simulink model "Commander_Stabilizer_Qdrone_wTrajTEMP"  (R2019a)
settings: Solver=ode2  StartTime=0.0  StopTime=inf  FixedStep=0.001  RelTol=1e-3  EnableMultiTasking=on
InitFcn:
  | set_param(gcs, 'ZoomFactor','FitSystem')
model workspace (MAT data in the model file):
  target_system = 1
undefined symbols (not defined in the file or in its folder): acc_calib, HIL
libraries: quarc_library x50, simulink x20, control_library x13, estimation_library x7
(part 3 of 3)

== matlab function Commander_Stabilizer_Qdrone_wTrajTEMP/Inner loop controller /inner loop MRFT subsytem/MRFT_NEW 1/MATLAB Function ==
  settings: updateMethod=DISCRETE
  data: err input; output output; beta input; h input; no_switch_delay_in_s input; num_of_peak_conf_samples input; sim_time input; e_max_o output; e_min_o output; sw_max_o output; sw_min_o output
% MRFT algorithm with false switching prevention mechanism
% June 2020
% Coded By M. Chehadeh, Khalifa University
function [output,e_max_o,e_min_o,sw_max_o,sw_min_o]  = MRFT(err,beta,h,no_switch_delay_in_s,num_of_peak_conf_samples,sim_time)
persistent switch_time;
persistent last_output;
persistent e_max;
persistent e_min;
persistent has_reached_min;
persistent has_reached_max;
persistent peak_conf_counter;
mode_of_operation=1;
% mode_of_operation=0 take last e_max or e_min
% mode_of_operation=1 take current e_max or e_min and mirror it

output=0;
e_max_o=0;
e_min_o=0;
sw_max_o=0;
sw_min_o=0;
if isempty(switch_time)
    switch_time = sim_time;
    peak_conf_counter=0;
    e_max=0;
    e_min=0;
    if (err>0)
        has_reached_max=true;
        has_reached_min=false;
        last_output=h;
    else
        has_reached_max=false;
        has_reached_min=true;
        last_output=-h;
    end
    output=last_output;
    return;  
end
output=last_output;
if (sim_time-switch_time<=no_switch_delay_in_s)
    e_min_o=e_min;
    e_max_o=e_max;
    return;
end

if (last_output<0)
    if (err<e_min)
        e_min=err;
        peak_conf_counter=0;
    else
        peak_conf_counter=peak_conf_counter+1;
        if (peak_conf_counter>=num_of_peak_conf_samples)
            has_reached_min=true;
            peak_conf_counter=0;
        end
        e_max=err;
    end
    if (mode_of_operation==0)
        sw_min=((e_max-e_min)/2)+e_min+beta*((e_max-e_min)/2);
    elseif (mode_of_operation==1)
        e_max_star=-e_min;
        sw_min=((e_max_star-e_min)/2)+e_min+beta*((e_max_star-e_min)/2);
    end
    sw_min_o=sw_min;
    if (has_reached_min)
        if (err>sw_min)
            output=h;
            switch_time=sim_time;
            has_reached_min=false;
        else
            output=last_output;
        end
    end
else
    if (err>e_max)
        e_max=err;
        peak_conf_counter=0;
    else
        peak_conf_counter=peak_conf_counter+1;
        if (peak_conf_counter>=num_of_peak_conf_samples)
            has_reached_max=true;
            peak_conf_counter=0;
        end
        e_min=err;
    end
    if (mode_of_operation==0)
        sw_max=e_max-((e_max-e_min)/2)-(beta*((e_max-e_min)/2));
    elseif (mode_of_operation==1)
        e_min_star=-e_max;
        sw_max=e_max-((e_max-e_min_star)/2)-(beta*((e_max-e_min_star)/2));
    end    
    sw_max_o=sw_max;
    if (has_reached_max)
        if (err<sw_max)
            output=-h;
            switch_time=sim_time;
            has_reached_max=false;
        else
            output=last_output;
        end
    end
end
e_min_o=e_min;
e_max_o=e_max;
last_output=output;

== matlab function Commander_Stabilizer_Qdrone_wTrajTEMP/Outer loop/MATLAB Function ==
  data: FSM_state input; HF_smoothed_commands output; HF_desired_state input; HF_current_state input; safety_threshold input; height_signals output
function [HF_smoothed_commands, height_signals] = fcn(FSM_state, HF_desired_state, HF_current_state, safety_threshold)

HF_desired_state = min(HF_desired_state, safety_threshold);
HF_desired_state = max(HF_desired_state, -safety_threshold);

HF_smoothed_commands = HF_desired_state;
switch FSM_state
    case 1
        HF_smoothed_commands = HF_current_state;
    case 2
        HF_smoothed_commands = HF_current_state;
    case 3
        delta_move = (HF_desired_state - HF_current_state);
        delta_move_norm = norm(delta_move);
        if delta_move_norm>0.2
            delta_move = 0.2 * delta_move / delta_move_norm;
        end
        HF_smoothed_commands = HF_current_state + delta_move;
    case 4
        delta_move = (HF_desired_state - HF_current_state);
        delta_move_norm = norm(delta_move);
        if delta_move_norm>0.2
            delta_move = 0.2 * delta_move / delta_move_norm;
        end
        HF_smoothed_commands = HF_current_state + delta_move;
    case 5
        HF_smoothed_commands = HF_desired_state;%HF_current_state + 0.2*(HF_desired_state - HF_current_state) / norm(HF_desired_state - HF_current_state);
    case 6
        HF_low_desired_state = HF_current_state;
        HF_low_desired_state(3) = 0.1;        
        delta_move = (HF_low_desired_state - HF_current_state);
        delta_move_norm = norm(delta_move);
        if delta_move_norm>0.1
            delta_move = 0.1 * delta_move / delta_move_norm;
        end
        HF_smoothed_commands = HF_current_state + delta_move;
    case 7
        HF_low_desired_state = HF_current_state;
        HF_low_desired_state(3) = 0.1;        
        delta_move = (HF_low_desired_state - HF_current_state);
        delta_move_norm = norm(delta_move);
        if delta_move_norm>0.2
            delta_move = 0.2 * delta_move / delta_move_norm;
        end
        HF_smoothed_commands = HF_current_state + delta_move;
    case 8
        
        HF_low_desired_state = HF_current_state;
        HF_low_desired_state(3) = 0.1;        
        delta_move = (HF_low_desired_state - HF_current_state);
        delta_move_norm = norm(delta_move);
        if delta_move_norm>0.2
            delta_move = 0.2 * delta_move / delta_move_norm;
        end
        HF_smoothed_commands = HF_current_state + delta_move;
    case 9        
        HF_low_desired_state = HF_desired_state;
        HF_low_desired_state(3) = 0.1;        
        delta_move = (HF_low_desired_state - HF_current_state);
        delta_move_norm = norm(delta_move);
        if delta_move_norm>0.2
            delta_move = 0.2 * delta_move / delta_move_norm;
        end
        HF_smoothed_commands = HF_current_state + delta_move;
end

height_signals = [HF_smoothed_commands(3), HF_current_state(3), safety_threshold(3), HF_desired_state(3)]';

== matlab function Commander_Stabilizer_Qdrone_wTrajTEMP/motor command mapper/Set commands/Red - Low Voltage Green - Armed Blue - Disarmed/MATLAB Function LED Color Assignment ==
  data: arm input; value output; low_battery input
function value = fcn(arm, low_battery)

if low_battery
    value = 1;
elseif arm
    value = 2;
else 
    value = 3;
end

== matlab function Commander_Stabilizer_Qdrone_wTrajTEMP/logic/FSM MONITOR/STATE MACHINE LOGIC ==
  data: E_Abort output; isArm output; pt_ARM_to_TAKEOFF_THROTTLE output; pt_TAKE_OFF_HEIGHT_TO_AUTOLAND output; pt_FLIGHT_TO_AUTOLAND output; current_state input; initializing input; health_issue input; peripheral input; low_battery input; trigger_1 input; trigger_2 input; E_abort input; net_throttle_at_trim input; net_throttle_close_to_zero input; ctrl_throttle_close_to_zero input; take_off_successful input; flying_too_low input; flying_too_high input; close_to_ground input; pt_TAKEOFF_THROTTLE_TO_TAKEOFF_HEIGHT output; pt_TAKE_OFF_HEIGHT_TO_FLIGHT output; pt_AUTOLAND_TO_DISABLE output; pt_EMERGENCY_STOP_TO_DISABLE output; pt_EMERGENCY_ABORT_TO_DISABLE output; Error output; stop_model output; sensor_failed input
function [E_Abort, isArm, pt_ARM_to_TAKEOFF_THROTTLE, pt_TAKE_OFF_HEIGHT_TO_AUTOLAND, pt_FLIGHT_TO_AUTOLAND, pt_TAKEOFF_THROTTLE_TO_TAKEOFF_HEIGHT, pt_TAKE_OFF_HEIGHT_TO_FLIGHT, pt_AUTOLAND_TO_DISABLE, pt_EMERGENCY_STOP_TO_DISABLE, pt_EMERGENCY_ABORT_TO_DISABLE, Error, stop_model]...
    = SM_logic(current_state, initializing, health_issue, peripheral, low_battery, trigger_1, trigger_2, E_abort,...
    net_throttle_at_trim, net_throttle_close_to_zero, ctrl_throttle_close_to_zero, take_off_successful, flying_too_low, flying_too_high, close_to_ground, sensor_failed)

% Programmatic Logic Block
%
% Logic for the FSM is generated here based on a variety of signals.
% Mostly, logic to programmatically trigger the transition to either a 
% natural next state, or an Error state, is generated here.
%
% v2.1 - 4th October, 2018
%
% INPUTS:
% -------
% current_state = previous state of the FSM-------------------------------------------------- (#)         [1]
% initializing = signal representing that the system is initializing (first 5s + buffer)- - - (bool)      [1]
% comm = communication signal representing MAVLINK connection-------------------------------- (bool)      [1]
% peripheral = signal representing joystick and optitrack connection- - - - - - - - - - - - - (bool)      [2]
% low_battery = signal representing low battery---------------------------------------------- (bool)      [1]
% trigger_1 = trigger representing ARM/DISARM - - - - - - - - - - - - - - - - - - - - - - - - (bool)      [1]
% trigger_2 = trigger representing TAKEOFF/AUTOLAND------------------------------------------ (bool)      [1]
% motors_not_spinning = signal representing the motors not spinning - - - - - - - - - - - - - (bool)      [1]
% net_throttle_at_trim = trim throttle for the application drone ---------------------------- (bool)      [1]
% net_throttle_close_to_zero = net throttle is close to zero in emergency stop mode - - - - - (bool)      [1]
% ctrl_throttle_close_to_zero = ctrl throttle is close to zero in emergency stop mode - - - - (bool)      [1]
% take_off_successful = signal representing whether drone has taken-off successfully -------- (bool)      [1]
% flying_too_low = signal representing whether the drone's height is below threshold and cmd- (bool)      [1]
% flying_too_high = signal representing whether the drone's height is above threshold-------- (bool)      [1]
% close_to_ground = signal representing whether the drone is close to the ground to autoland- (bool)      [1]
% 
% OUTPUTS:
% --------
% Error = Whether an Error is issued or not                                                             (bool)    [1]
% E_Abort = fed through for ease of understanding flow (see STATE MACHINE TRANSITION BLOCK)             (bool)    [1]
% isArm = programmatic transition state                                                                 (bool)    [1]
% pt_ARM_to_TAKEOFF_THROTTLE = programmatic transition state BEGIN_STATE_TO_FINAL_STATE                 (bool)    [1]
% pt_TAKEOFF_THROTTLE_TO_TAKEOFF_HEIGHT = programmatic transition state BEGIN_STATE_TO_FINAL_STATE      (bool)    [1]
% pt_TAKE_OFF_HEIGHT_TO_AUTOLAND = programmatic transition state BEGIN_STATE_TO_FINAL_STATE             (bool)    [1]
% pt_TAKEOFF_THROTTLE_TO_TAKEOFF_HEIGHT = programmatic transition state BEGIN_STATE_TO_FINAL_STATE      (bool)    [1]
% pt_TAKE_OFF_HEIGHT_TO_FLIGHT = programmatic transition state BEGIN_STATE_TO_FINAL_STATE               (bool)    [1]
% pt_AUTOLAND_TO_DISABLE = programmatic transition state BEGIN_STATE_TO_FINAL_STATE                     (bool)    [1]
% pt_EMERGENCY_STOP_TO_DISABLE = programmatic transition state BEGIN_STATE_TO_FINAL_STATE               (bool)    [1]
% pt_EMERGENCY_ABORT_TO_DISABLE = programmatic transition state BEGIN_STATE_TO_FINAL_STATE              (bool)    [1]
% stop_model = STOP THE MODEL AFTER                                                                     (bool)    [1]

Error = 0;
E_Abort = E_abort;
isArm = false;
pt_ARM_to_TAKEOFF_THROTTLE = false;
pt_TAKEOFF_THROTTLE_TO_TAKEOFF_HEIGHT = false;
pt_TAKE_OFF_HEIGHT_TO_AUTOLAND = false;
pt_TAKE_OFF_HEIGHT_TO_FLIGHT = false;
pt_FLIGHT_TO_AUTOLAND = false;
pt_AUTOLAND_TO_DISABLE = false;
pt_EMERGENCY_STOP_TO_DISABLE = false;
pt_EMERGENCY_ABORT_TO_DISABLE = false;
stop_model = 0;

switch current_state
    %---------------------------------------------------------------------%
    case 1 % IDLE STATE
        if (health_issue)||... % mavlink issue
           (peripheral(1))||... % joystick issue
           (peripheral(2))||... % optitrack issue
           ((trigger_1)&&(initializing))||... % armed while initializing
           (trigger_2)||... % tried to takeoff
           (sensor_failed)||... % if sensor (IMU) failure is detected on drone stabilizer
           (~ctrl_throttle_close_to_zero)||... % if throttle isn't at zero, don't arm
           (low_battery) % low battery
           %----------------------------------------%
            Error = 1;
        elseif trigger_1 % user arms
            isArm = true;
        end
    %---------------------------------------------------------------------%    
    case 2 % ARMED STATE
        isArm = trigger_1;
        if (health_issue)||... % mavlink issue
           (peripheral(1))||... % joystick issue
           (peripheral(2))||... % optitrack issue
           (low_battery)||... % low battery
           (~ctrl_throttle_close_to_zero)||... % if throttle isn't at zero, don't arm
           (sensor_failed) % if sensor (IMU) failure is detected on drone stabilizer
           %----------------------------------------%
            Error = 1;
        elseif trigger_1 && trigger_2
            pt_ARM_to_TAKEOFF_THROTTLE = true;
        end        
    %---------------------------------------------------------------------%
    case 3 % TAKEOFF_THROTTLE STATE
        if (health_issue)||... % mavlink issue
           (peripheral(1))||... % joystick issue
           (peripheral(2))||... % optitrack issue
           (low_battery)||... % low battery
           (~trigger_1)||... % user disarms
           (~trigger_2)||... % user commands auto-land before drone starts taking off
           (sensor_failed)%||... % if sensor (IMU) failure is detected on drone stabilizer
           %(~ctrl_throttle_close_to_zero) % if throttle isn't at zero, don't arm
           %----------------------------------------%
            Error = 1;
        elseif net_throttle_at_trim
            pt_TAKEOFF_THROTTLE_TO_TAKEOFF_HEIGHT = true;
        end
    %---------------------------------------------------------------------%
    case 4 % TAKEOFF_HEIGHT STATE
        if (health_issue)||... % mavlink issue
           (peripheral(1))||... % joystick issue
           (peripheral(2))||... % optitrack issue
           (~trigger_1)||... % user disarms
           (sensor_failed)||... % if sensor (IMU) failure is detected on drone stabilizer
           (flying_too_high)
           %(flying_too_low)||... % current height is below safety threshold but 
           %...                   % commanded height is not
           
            %----------------------------------------%
            Error = 1;
        elseif (~trigger_2)||low_battery
            pt_TAKE_OFF_HEIGHT_TO_AUTOLAND = true;
        elseif take_off_successful
            pt_TAKE_OFF_HEIGHT_TO_FLIGHT = true;
        end
    %---------------------------------------------------------------------%
    case 5 % FLIGHT STATE
        if (health_issue)||... % mavlink issue
           (peripheral(1))||... % joystick issue
           (peripheral(2))||... % optitrack issue
           (~trigger_1)||... % user disarms
           (flying_too_low)||... % current height is below safety threshold but 
           ...                   % commanded height is not
           (sensor_failed)||... % if sensor (IMU) failure is detected on drone stabilizer
           (flying_too_high) % flying above safety margin (w.r.t optitrack)
           %----------------------------------------%
            Error = 1;
        elseif (~trigger_2)||low_battery
            pt_FLIGHT_TO_AUTOLAND = true;
        end
    %---------------------------------------------------------------------%
    case 6 % AUTOLAND STATE
        if (health_issue)||... % mavlink issue
           (peripheral(1))||... % joystick issue
           (peripheral(2))||... % optitrack issue
           (~trigger_1)||... % user disarms
           (trigger_2)||... % user tries to takeoff while landing
           (sensor_failed)||... % if sensor (IMU) failure is detected on drone stabilizer
           (flying_too_high) % flying above safety margin (w.r.t optitrack)
           %----------------------------------------%
            Error = 1;
        elseif close_to_ground 
            pt_AUTOLAND_TO_DISABLE = true;
        end
    %---------------------------------------------------------------------%
    case 7 % EMERGENCY LAND STATE
        if net_throttle_close_to_zero 
            pt_EMERGENCY_STOP_TO_DISABLE = true;
        end
    %---------------------------------------------------------------------%
    case 8 % EMERGENCY ABORT STATE
        pt_EMERGENCY_ABORT_TO_DISABLE = true;
    %---------------------------------------------------------------------%
    case 9
        % Stop the model.
        stop_model = 1;
end

== matlab function Commander_Stabilizer_Qdrone_wTrajTEMP/logic/FSM MONITOR/STATE MACHINE TRANSITION ==
  data: current_state input; E_Abort input; isArm input; pt_ARM_to_TAKEOFF_THROTTLE input; pt_TAKE_OFF_HEIGHT_TO_AUTOLAND input; pt_FLIGHT_TO_AUTOLAND input; Next_state output; pt_TAKEOFF_THROTTLE_TO_TAKEOFF_HEIGHT input; pt_TAKE_OFF_HEIGHT_TO_FLIGHT input; pt_AUTOLAND_TO_DISABLE input; pt_EMERGENCY_STOP_TO_DISABLE input; pt_EMERGENCY_ABORT_TO_DISABLE input; Error input
function Next_state = SM_transition(current_state, E_Abort, isArm, pt_ARM_to_TAKEOFF_THROTTLE, pt_TAKE_OFF_HEIGHT_TO_AUTOLAND, pt_FLIGHT_TO_AUTOLAND, pt_TAKEOFF_THROTTLE_TO_TAKEOFF_HEIGHT, pt_TAKE_OFF_HEIGHT_TO_FLIGHT, pt_AUTOLAND_TO_DISABLE, pt_EMERGENCY_STOP_TO_DISABLE, pt_EMERGENCY_ABORT_TO_DISABLE, Error)

% Programmatic Transition Block
%
% FINITE STATE MACHINE (FSM) with 9 states as described below, transitioning based on the 
% values of the isArm, transition signals, Error, and E_Abort
%
% v2.1 - 4th October, 2018
%
% INPUTS:
% ------
% current_state = Current state of the FSM        (#)     [1]
% E_Abort                                         (bool)  [1]
% isArm                                           (bool)  [1]
% pt_ARM_TO_TAKEOFF_THROTTLE                      (bool)  [1]
% pt_TAKE_OFF_HEIGHT_TO_AUTOLAND                  (bool)  [1]
% pt_FLIGHT_TO_AUTOLAND                           (bool)  [1]
% pt_TAKEOFF_THROTTLE_TO_TAKEOFF_HEIGHT           (bool)  [1]
% pt_TAKE_OFF_HEIGHT_TO_FLIGHT                    (bool)  [1]
% pt_AUTOLAND_TO_DISABLE                          (bool)  [1]
% pt_EMERGENCY_STOP_TO_DISABLE                    (bool)  [1]
% pt_EMERGENCY_ABORT_TO_DISABLE                   (bool)  [1]
% Error                                           (bool)  [1]
%
% OUTPUT:
% -------
% Next_state = Next state of the FSM              (#)     [1]

Next_state = double(0);
switch current_state
%-------------------------------------------------------------------------%
    case 1 % IDLE STATE
        if E_Abort
            Next_state = 8; % GOTO EMERGENCY ABORT STATE
        elseif Error
            Next_state = 7; % GOTO EMERGENCY STOP STATE
        elseif isArm
            Next_state = 2; % GOTO ARMED STATE
        else
            Next_state = 1; % STAY IN IDLE STATE
        end
%-------------------------------------------------------------------------%
    case 2 % ARMED STATE
        if E_Abort
            Next_state = 8; % GOTO EMERGENCY ABORT STATE
        elseif Error
            Next_state = 7; % GOTO EMERGENCY STOP STATE
        elseif ~isArm
            Next_state = 1; % GOTO IDLE STATE
        elseif pt_ARM_to_TAKEOFF_THROTTLE
            Next_state = 3; % GOTO TAKEOFF_THROTTLE STATE 
        else
            Next_state = 2; % STAY IN ARMED STATE
        end
%-------------------------------------------------------------------------%
    case 3 % TAKEOFF_THROTTLE STATE
        if E_Abort
            Next_state = 8; % GOTO EMERGENCY ABORT STATE
        elseif Error
            Next_state = 7; % GOTO EMERGENCY STOP STATE
        elseif pt_TAKEOFF_THROTTLE_TO_TAKEOFF_HEIGHT
            Next_state = 4; % GOTO TAKEOFF_HEIGHT STATE
        else
            Next_state = 3; % STAY IN TAKEOFF_THROTTLE STATE
        end
%-------------------------------------------------------------------------%
    case 4 % TAKEOFF_HEIGHT STATE
        if E_Abort
            Next_state = 8; % GOTO EMERGENCY ABORT STATE
        elseif Error
            Next_state = 7; % GOTO EMERGENCY STOP STATE
        elseif pt_TAKE_OFF_HEIGHT_TO_AUTOLAND
            Next_state = 6;
        elseif pt_TAKE_OFF_HEIGHT_TO_FLIGHT
            Next_state = 5; % GOTO FLIGHT STATE
        else
            Next_state = 4; % STAY IN TAKEOFF_HEIGHT STATE
        end
%-------------------------------------------------------------------------%
    case 5 % FLIGHT STATE
        if E_Abort
            Next_state = 8; % GOTO EMERGENCY ABORT STATE
        elseif Error
            Next_state = 7; % GOTO EMERGENCY STOP STATE
        elseif pt_FLIGHT_TO_AUTOLAND
            Next_state = 6; % GOTO AUTO_LAND STATE
        else
            Next_state = 5; % STAY IN FLIGHT STATE
        end
%-------------------------------------------------------------------------%       
    case 6 % AUTO_LAND STATE
        if E_Abort
            Next_state = 8; % GOTO EMERGENCY ABORT STATE
        elseif Error
            Next_state = 7; % GOTO EMERGENCY STOP STATE
        elseif pt_AUTOLAND_TO_DISABLE
            Next_state = 9; % GOTO DISABLE STATE
        else
            Next_state = 6; % STAY IN AUTO_LAND STATE
        end
%-------------------------------------------------------------------------%
    case 7 % EMERGENCY STOP STATE
        if E_Abort
            Next_state = 8; % GOTO EMERGENCY ABORT STATE
        elseif pt_EMERGENCY_STOP_TO_DISABLE
            Next_state = 9; % GOTO DISABLE STATE
        else
            Next_state = 7; % STAY IN EMERGENCY STOP STATE
        end
%-------------------------------------------------------------------------%
    case 8 % EMERGENCY ABORT
        if pt_EMERGENCY_ABORT_TO_DISABLE
            Next_state = 9; % GOTO DISABLE STATE
        else 
            Next_state = 8; % STAY IN EMERGENCY ABORT STATE
        end
%-------------------------------------------------------------------------%    
    case 9 % DISABLE
        Next_state = 9; % Always stay in DISABLE state if you are here    
end

== matlab function Commander_Stabilizer_Qdrone_wTrajTEMP/Pull Detector1/MATLAB Function ==
  settings: updateMethod=DISCRETE  sampleTime=0.001
  data: error_z input; acc_x input; acc_y input; acc_z input; roll input; pitch input; yaw input; detection_output output
function detection_output  = LSTM(error_z, acc_x, acc_y, acc_z, roll, pitch, yaw)

persistent drone_handover_model
persistent p_01_h_t
persistent p_01_c_t
persistent p_03_h_t
persistent p_03_c_t
persistent scaling_params
persistent buffer
persistent counter
persistent clean_detection

downsample_by = 5;

if isempty(drone_handover_model)
    drone_handover_model = coder.load('Model_2f_norm/drone_handover_model.mat');
    scaling_params = coder.load('Model_2f_norm/Scaling.mat');
    p_01_h_t = single(zeros(1,200));
    p_01_c_t = single(randn(1,200)/10);
    p_03_h_t = single(zeros(1,100));
    p_03_c_t = single(randn(1,100)/10);
    buffer = single(zeros(7,downsample_by));
    counter = 1;
    clean_detection = 0;
end

buffer(1,counter) = error_z;
buffer(2,counter) = acc_x;
buffer(3,counter) = acc_y;
buffer(4,counter) = acc_z;
buffer(5,counter) = roll;
buffer(6,counter) = pitch;
buffer(7,counter) = yaw;

if counter == 5
    counter = 1;
    error_z = mean(buffer(1,:));
    acc_x = mean(buffer(2,:));
    acc_y = mean(buffer(3,:));
    acc_z = mean(buffer(4,:));
    roll = mean(buffer(5,:));
    pitch = mean(buffer(6,:));
    yaw = mean(buffer(7,:));
    % 
    [acc_x_inertial, acc_y_inertial, acc_z_inertial] = R_B2I(roll, pitch, yaw, acc_x, acc_y, acc_z);
    % 
    l2_norm_acc_inertial = sqrt(acc_x_inertial.^2 + acc_y_inertial.^2);
    % 
    % [ori_body_x, ori_body_y, ori_body_z] = R_I2B(roll, pitch, yaw, 0, 0, 1);
    % 
%     l2_norm_ori = sqrt(ori_body_x.^2 + ori_body_y.^2);
%     % 
%     acc_dir = atan2(acc_y_inertial, acc_x_inertial);
%     ori_dir = atan2(ori_body_y, ori_body_x);
%     
%     if abs(acc_dir - ori_dir) <= pi
%         dist_acc_ori = abs(acc_dir - ori_dir);
%     else
%         dist_acc_ori = 2*pi - abs(acc_dir - ori_dir);
%     end
    
    % %%Scaling
    % % X_std = (X - X.min(axis=0)) / (X.max(axis=0) - X.min(axis=0))
    error_z = (error_z - scaling_params.data_Z_params(1)) / (scaling_params.data_Z_params(2)-scaling_params.data_Z_params(1));
    error_z = error_z * 2 - 1;
    l2_norm_acc_inertial = (l2_norm_acc_inertial  - scaling_params.data_L2_norm_inertial_params(1)) / (scaling_params.data_L2_norm_inertial_params(2)-scaling_params.data_L2_norm_inertial_params(1));
    l2_norm_acc_inertial = l2_norm_acc_inertial * 2 - 1;
    %     l2_norm_ori = (l2_norm_ori - scaling_params.data_L2_norm_ori_params(1)) / (scaling_params.data_L2_norm_ori_params(2)-scaling_params.data_L2_norm_ori_params(1));
%     dist_acc_ori = (dist_acc_ori - scaling_params.data_dist_acc_ori_params(1)) / (scaling_params.data_dist_acc_ori_params(2)-scaling_params.data_dist_acc_ori_params(1));
    % 

    input_data = [error_z l2_norm_acc_inertial];

    [detection, p_01_c_t, p_01_h_t, p_03_c_t, p_03_h_t] = model_classify(input_data, ...
                                                                         drone_handover_model, ...
                                                                         p_01_c_t, ...
                                                                         p_01_h_t, ...
                                                                         p_03_c_t, ...
                                                                         p_03_h_t);
                                                                     
    clean_detection = clean(detection, 0.5);
%     clean_detection = double(detection);
end

counter = counter + 1;

% dist_acc_ori_out = dist_acc_ori;
% l2_norm_ori_out = l2_norm_ori;
% l2_norm_acc_out = l2_norm_acc_inertial;
detection_output = double(clean_detection);

% function [detection_output, error_output, l2_output] = LSTM_offline(error_z_, l2_norm_acc_inertial_)
% 
% persistent drone_handover_model
% persistent p_01_h_t
% persistent p_01_c_t
% persistent p_03_h_t
% persistent p_03_c_t
% persistent scaling_params
% persistent buffer
% persistent counter
% persistent clean_detection
% 
% downsample_by = 5;
% 
% if isempty(drone_handover_model)
%     drone_handover_model = coder.load('Model_2f_norm/drone_handover_model.mat');
%     p_01_h_t = single(zeros(1,200));
%     p_01_c_t = single(randn(1,200)/10);
%     p_03_h_t = single(zeros(1,100));
%     p_03_c_t = single(randn(1,100)/10);
%     buffer = single(zeros(7,downsample_by));
%     counter = 1;
%     clean_detection = 0;
% end
% 
% 
% input_data = [error_z_ l2_norm_acc_inertial_];
% 
% [detection, p_01_c_t, p_01_h_t, p_03_c_t, p_03_h_t] = model_classify(input_data, ...
%                                                                      drone_handover_model, ...
%                                                                      p_01_c_t, ...
%                                                                      p_01_h_t, ...
%                                                                      p_03_c_t, ...
%                                                                      p_03_h_t);
% 
% clean_detection = clean(detection, 0.5);
% 
% error_output = error_z_;
% l2_output = l2_norm_acc_inertial_;
% detection_output = double(clean_detection);

== matlab function Commander_Stabilizer_Qdrone_wTrajTEMP/Pull Detector1/MATLAB Function1 ==
  settings: updateMethod=DISCRETE  sampleTime=0.001
  data: u input; y output; threshold input
function y = prediction_filter(u, threshold)

persistent counter_ones
persistent counter_zeros
persistent pull_detected
persistent prev_u

if isempty(counter_ones)
    counter_ones = 0;
    counter_zeros = 0;
    prev_u = 0;
end

if u == 1
    counter_ones = counter_ones + 1;
else
    counter_zeros = counter_zeros + 1;     
end

if prev_u == 0 && u == 1
    counter_zeros = 0;
end

if counter_ones > threshold && counter_zeros < threshold
    pull_detected = 1;
else
    pull_detected = 0;
end

if counter_zeros >= threshold
    counter_ones = 0;
end

prev_u = double(u);
y = pull_detected;

== matlab function Commander_Stabilizer_Qdrone_wTrajTEMP/Inner loop controller /inner loop MRFT subsytem/MRFT_NEW /MATLAB Function ==
  settings: updateMethod=DISCRETE
  data: err input; output output; beta input; h input; no_switch_delay_in_s input; num_of_peak_conf_samples input; sim_time input; e_max_o output; e_min_o output; sw_max_o output; sw_min_o output
% MRFT algorithm with false switching prevention mechanism
% June 2020
% Coded By M. Chehadeh, Khalifa University
function [output,e_max_o,e_min_o,sw_max_o,sw_min_o]  = MRFT(err,beta,h,no_switch_delay_in_s,num_of_peak_conf_samples,sim_time)
persistent switch_time;
persistent last_output;
persistent e_max;
persistent e_min;
persistent has_reached_min;
persistent has_reached_max;
persistent peak_conf_counter;
mode_of_operation=1;
% mode_of_operation=0 take last e_max or e_min
% mode_of_operation=1 take current e_max or e_min and mirror it

output=0;
e_max_o=0;
e_min_o=0;
sw_max_o=0;
sw_min_o=0;
if isempty(switch_time)
    switch_time = sim_time;
    peak_conf_counter=0;
    e_max=0;
    e_min=0;
    if (err>0)
        has_reached_max=true;
        has_reached_min=false;
        last_output=h;
    else
        has_reached_max=false;
        has_reached_min=true;
        last_output=-h;
    end
    output=last_output;
    return;  
end
output=last_output;
if (sim_time-switch_time<=no_switch_delay_in_s)
    e_min_o=e_min;
    e_max_o=e_max;
    return;
end

if (last_output<0)
    if (err<e_min)
        e_min=err;
        peak_conf_counter=0;
    else
        peak_conf_counter=peak_conf_counter+1;
        if (peak_conf_counter>=num_of_peak_conf_samples)
            has_reached_min=true;
            peak_conf_counter=0;
        end
        e_max=err;
    end
    if (mode_of_operation==0)
        sw_min=((e_max-e_min)/2)+e_min+beta*((e_max-e_min)/2);
    elseif (mode_of_operation==1)
        e_max_star=-e_min;
        sw_min=((e_max_star-e_min)/2)+e_min+beta*((e_max_star-e_min)/2);
    end
    sw_min_o=sw_min;
    if (has_reached_min)
        if (err>sw_min)
            output=h;
            switch_time=sim_time;
            has_reached_min=false;
        else
            output=last_output;
        end
    end
else
    if (err>e_max)
        e_max=err;
        peak_conf_counter=0;
    else
        peak_conf_counter=peak_conf_counter+1;
        if (peak_conf_counter>=num_of_peak_conf_samples)
            has_reached_max=true;
            peak_conf_counter=0;
        end
        e_min=err;
    end
    if (mode_of_operation==0)
        sw_max=e_max-((e_max-e_min)/2)-(beta*((e_max-e_min)/2));
    elseif (mode_of_operation==1)
        e_min_star=-e_max;
        sw_max=e_max-((e_max-e_min_star)/2)-(beta*((e_max-e_min_star)/2));
    end    
    sw_max_o=sw_max;
    if (has_reached_max)
        if (err<sw_max)
            output=-h;
            switch_time=sim_time;
            has_reached_max=false;
        else
            output=last_output;
        end
    end
end
e_min_o=e_min;
e_max_o=e_max;
last_output=output;

== matlab function Commander_Stabilizer_Qdrone_wTrajTEMP/Communication1/Detect Communication Loss/MATLAB Function ==
  settings: updateMethod=DISCRETE
  data: time input; stream_connection_loss output; state input; error input; ms_time input; data_loss output
function [stream_connection_loss , data_loss] = fcn(time, state, error, ms_time)

persistent ms_time_prev
    if isempty(ms_time_prev)
        ms_time_prev = 0;
    end

stream_connection_loss = 0;
data_loss = 0;
if time > 3
    if ((state ~= 2)&&(error < 0))
        % stream connection is not established correctly
        stream_connection_loss = 1;
    end

    if (ms_time == ms_time_prev)&&(ms_time > 0)
        % data is stale
        data_loss = 1;
    end
end

ms_time_prev = ms_time;
